simulink model "untitled3"  (R2023a)
settings: Solver=VariableStepAuto  StartTime=0.0  StopTime=10.0  RelTol=1e-3
settings Model: Creator=User  LastModifiedBy=User

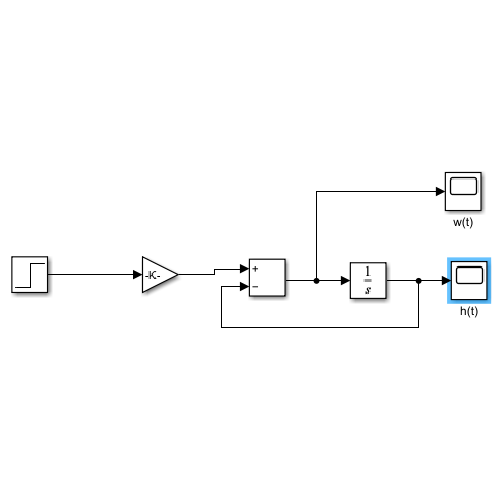
[thumbnail: Simulink's stored preview of the top-level diagram]
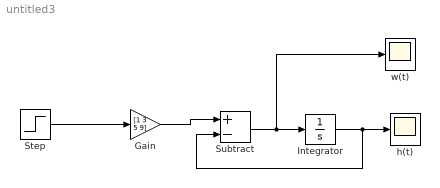
== system untitled3 ==
  Gain : Gain  Gain=[1 3 5 9]
  Integrator : Integrator
  Step : Step  SampleTime=0
  Subtract : Sum  Inputs=+-
  h(t) : Scope
  w(t) : Scope
  wires:
  Step/1 -> Gain/1
  Gain/1 -> Subtract/1
  Subtract/1 -> w(t)/1, Integrator/1
  Integrator/1 -> Subtract/2, h(t)/1
